simulink model "main_RI_LIEKF"  (R2023a)
settings: Solver=FixedStepAuto  StartTime=0.0  StopTime=220  FixedStep=0.01  RelTol=1e-3
InitFcn:
  | initNavigation0612_AOA;
values from neighbouring files (symbols this model uses):
  CF_enable = 0    [initNavigation.m]
  dt = 0.01    [initNavigation.m]
  dtDelay = -0.03    [initNavigation.m]
  g0 = 9.795    [initNavigation.m]
  gam0_rad = 0/57.3    (= 0)    [initNavigation.m]
  H_sensor_type = 0    [initNavigation.m]
  KF_enable = 1    [initNavigation.m]
  P0 = diag([1*ones(3,1);0.01*ones(3,1);0.1*ones(3,1);0.001*ones(3,1);0.00001*ones(3,1)])    [initNavigation.m]
  P0_RIEKF = diag([1*ones(3,1);0.01*ones(3,1);0.1*ones(3,1);0.001*ones(3,1);0.00001*ones(3,1);      0.01*ones(3,1);[0;2;2]/57.3;[0.1;0.1;0.1]])^2    [initNavigation.m]
  pd0 = 0    [initNavigation.m]
  pe0 = 0    [initNavigation.m]
  phi0_rad = 0/57.3    (= 0)    [initNavigation.m]
  pn0 = 0    [initNavigation.m]
  psi = -178    [initNavigation.m]
  psi0_rad = 0/57.3    (= 0)    [initNavigation.m]
  state_dim = 24    [initNavigation.m]
  Time = 0:0.01:(size(traindata.AttackAngle,1) - 1)*0.01    [NNLiftCoefficientFit.m]
  vd0 = 0    [initNavigation.m]
  ve0 = 0    [initNavigation.m]
  vn0 = 0    [initNavigation.m]
undefined symbols (not defined in the file or in its folder): DiscIntNeverNeededParam, Discrete, INS_CONST, INS_EXPORT, INS_PARAM, magnitude, p, param, pInitialization, sys
libraries: simulink x69, simulink_extras x64, dspstat3 x56, sharedtransform x49, ctrlSharedLib x36, sharedTrackingLibrary x17, FMT_Model_Lib x13, matrix_library x12, deeplib x4, dspsolvers x4, vrlib x4, aerolibconvert2 x1
(part 8 of 22)

== system main_RI_LIEKF/State estimation/0609bk/INS propogation/Init_PVQ ==
  QGC_sensor_reinit : Inport
  accl_B_m/s2_LPF : Inport  Port=2
  Magn_B_guess_LPF : Inport  Port=3
  pos_NED : Inport  Port=4
  vel_NED : Inport  Port=5
  Constant : Constant  Value=[1 0 0 0]  OutDataTypeStr=single
  Constant1 : Constant  OutDataTypeStr=uint8
  Constant2 : Constant  Value=[0;0;0]  OutDataTypeStr=single
  Constant3 : Constant  Value=[0;0;0]  OutDataTypeStr=single
  Detect Increase : simulink/Logic and Bit Operations/Detect Increase  vinit=0.0  OutDataTypeStr=boolean
  Horizontal_attitude : Subsystem  TreatAsAtomicUnit=on
  Memory : Memory
  Scope : Scope  NumInputPorts=2
  Scope1 : Scope
  Scope2 : Scope
  Subsystem : Subsystem
  Subsystem1 : Subsystem
  Switch{,1..3} (4 alike) : Switch  Criteria=u2 > Threshold  SaturateOnIntegerOverflow=off  InputSameDT=off
  quat_0 : Outport
  v0 : Outport  Port=2
  p0 : Outport  Port=3
  wires:
  vel_NED/1 -> Switch2/1
  pos_NED/1 -> Switch3/1
  Switch3/1 -> p0/1
  Switch2/1 -> v0/1
  Constant3/1 -> Switch3/3
  Constant2/1 -> Switch2/3
  Detect Increase/1 -> Scope/2, Switch1/2, Horizontal_attitude/Enable
  Magn_B_guess_LPF/1 -> Subsystem1/1(data)
  QGC_sensor_reinit/1 -> Scope/1, Detect Increase/1
  accl_B_m/s2_LPF/1 -> Subsystem/1(data)
  Switch1/1 -> Scope1/1, Switch/2, Switch3/2, Switch2/2, Memory/1
  Constant1/1 -> Switch1/1
  Constant/1 -> Switch/3
  Horizontal_attitude/1(quat_0) -> Switch/1
  Switch/1 -> Scope2/1, quat_0/1
  Memory/1 -> Switch1/3
  Subsystem/1(mean_data) -> Horizontal_attitude/1(accl_mean_B_m/s_LPF)
  Subsystem1/1(mean_data) -> Horizontal_attitude/2(Magn_mean_B_guess_LPF)

== system main_RI_LIEKF/State estimation/0609bk/INS propogation/att_update ==
  Rbn : Inport
  gyro : Inport  Port=2
  quat_0 : Inport  Port=3  PortDimensions=4
  init_flag : Inport  Port=4
  Bus Creator1 : BusCreator  Inputs=1
  Constant : Constant  Value=dt
  Data Type Conversion : DataTypeConversion  OutDataTypeStr=single  SaturateOnIntegerOverflow=off  RndMeth=Floor
  Delay1 : Delay  DelayLength=1  InitialConditionSource=Input port  InitialCondition=0  ExternalReset=Level hold
      settings: InputPortMap=u0,r5,p4
  Detect Increase : simulink/Logic and Bit Operations/Detect Increase  vinit=0.0  OutDataTypeStr=boolean
  MATLAB Function : MATLAB Function  TreatAsAtomicUnit=on
  Quaternions to Direction Cosine Matrix : sharedtransform/Quaternions to  Direction Cosine Matrix  aMode=aMode
      settings: LibrarySourceBlock=|
      | aerolibtransform2/Quaternions to
      | Direction Cosine Matrix
  Transpose : Math  Operator=transpose
  att_update1 : Outport
  wires:
  init_flag/1 -> Detect Increase/1
  quat_0/1 -> Quaternions to Direction Cosine Matrix/1
  gyro/1 -> MATLAB Function/2(w)  "w"
  Constant/1 -> MATLAB Function/3(dt)
  Quaternions to Direction Cosine Matrix/1 -> Transpose/1
  Transpose/1 -> Delay1/3
  Delay1/1 -> MATLAB Function/1(Rbn_k_1)
  Detect Increase/1 -> Delay1/2
  Bus Creator1/1 -> att_update1/1
  MATLAB Function/1(Rbn) -> Data Type Conversion/1  "DCM_b_n"
  Rbn/1 -> Delay1/1
  Data Type Conversion/1 -> Bus Creator1/1  "DCM_b_n"

== system main_RI_LIEKF/State estimation/0609bk/INS propogation/vel_pos_update ==
  <DCM_b_n> : Inport
  Ab : Inport  Port=2
  v0 : Inport  Port=3
  p0 : Inport  Port=4
  QGC_init : Inport  Port=5
  pn : Inport  Port=6
  vn : Inport  Port=7
  Kinematic Equation : Subsystem
  QGC_init1 : InportShadow  Port=5
  pos update : Subsystem
  vel update : Subsystem
  p_k : Outport
  V : Outport  Port=2
  wires:
  QGC_init1/1 -> pos update/3(QGC_init)
  pos update/1(p_k) -> p_k/1
  p0/1 -> pos update/4(p0)
  pn/1 -> pos update/2(pn)
  v0/1 -> vel update/4(v0)
  vn/1 -> vel update/3(vn)
  Kinematic Equation/1(An) -> vel update/2(An)
  QGC_init/1 -> vel update/1(QGC_init)
  Ab/1 -> Kinematic Equation/2(Ab)
  <DCM_b_n>/1 -> Kinematic Equation/1(Cbn)
  vel update/1(vel_k) -> V/1, pos update/1(vel_k)

== system main_RI_LIEKF/State estimation/15dim KF1/Error State Kalman Filter/Cal Phi ==
  <DCM_b_n> : Inport
  wxyz : Inport  Port=2
  axyz : Inport  Port=3
  Constant : Constant  Value=dt
  MATLAB Function1 : MATLAB Function  TreatAsAtomicUnit=on
  Transpose : Math  Operator=transpose
  Phi : Outport
  wires:
  Transpose/1 -> MATLAB Function1/2(Cnb)
  Constant/1 -> MATLAB Function1/4(dt)
  axyz/1 -> MATLAB Function1/1(axyz)
  wxyz/1 -> MATLAB Function1/3(wxyz)
  MATLAB Function1/1(Phi) -> Phi/1
  <DCM_b_n>/1 -> Transpose/1

== system main_RI_LIEKF/State estimation/15dim KF1/Error State Kalman Filter/Cal Q ==
  <DCM_b_n> : Inport
  wxyz : Inport  Port=2
  Constant : Constant  Value=dt
  MATLAB Function1 : MATLAB Function  TreatAsAtomicUnit=on
  Transpose : Math  Operator=transpose
  Qd : Outport
  wires:
  Transpose/1 -> MATLAB Function1/1(Cnb)
  Constant/1 -> MATLAB Function1/3(dt)
  <DCM_b_n>/1 -> Transpose/1
  MATLAB Function1/1(Qd) -> Qd/1
  wxyz/1 -> MATLAB Function1/2(wxyz)

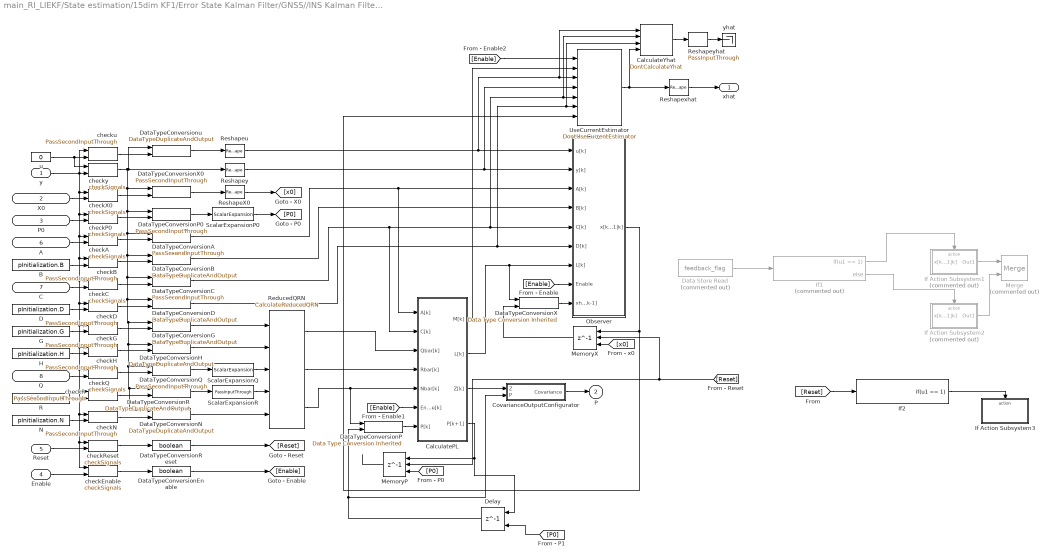
== system main_RI_LIEKF/State estimation/15dim KF1/Error State Kalman Filter/GNSS//INS Kalman Filter1 ==
  y : Inport
  X0 : Inport  Port=2
  P0 : Inport  Port=3
  Enable : Inport  Port=4
  Reset : Inport  Port=5
  A : Inport  Port=6
  C : Inport  Port=7
  Q : Inport  Port=8
  B : Constant  Value=pInitialization.B  VectorParams1D=off  OutDataTypeStr=Inherit: Inherit via back propagation
  CalculatePL : Subsystem  AncestorBlock=ctrlSharedLib/KalmanFilterUtilities/DTCalculatePL  TreatAsAtomicUnit=on  SystemSampleTime=pInitialization.Ts  mask(ctrlKalmanFilterDTCalculatePL){}
      settings: LibrarySourceBlock=ctrlSharedLib/KalmanFilterUtilities/DTCalculatePL
  CalculateYhat : ctrlSharedLib/KalmanFilterUtilities/DontCalculateYhat  SystemSampleTime=-1  VariantActivationTime=update diagram  Latency=0  AutoFrameSizeCalculation=off
  CovarianceOutputConfigurator : Subsystem
  D : Constant  Value=pInitialization.D  VectorParams1D=off  OutDataTypeStr=Inherit: Inherit via back propagation
  Data Store Read : DataStoreRead  Commented=on  DataStoreName=feedback_flag  IndexOptions=Index vector (dialog)  Indices=1  OutputSizes=1
  DataTypeConversionA : ctrlSharedLib/KalmanFilterUtilities/PassSecondInputThrough  SystemSampleTime=-1  VariantActivationTime=update diagram  Latency=0  AutoFrameSizeCalculation=off
  DataTypeConversionB : ctrlSharedLib/Utilities/DataTypeDuplicateAndOutput  SystemSampleTime=-1  VariantActivationTime=update diagram  Latency=0  AutoFrameSizeCalculation=off
  DataTypeConversionC : ctrlSharedLib/KalmanFilterUtilities/PassSecondInputThrough  SystemSampleTime=-1  VariantActivationTime=update diagram  Latency=0  AutoFrameSizeCalculation=off
  DataTypeConversionD : ctrlSharedLib/Utilities/DataTypeDuplicateAndOutput  SystemSampleTime=-1  VariantActivationTime=update diagram  Latency=0  AutoFrameSizeCalculation=off
  DataTypeConversionEnable : DataTypeConversion  OutDataTypeStr=boolean  SaturateOnIntegerOverflow=off  RndMeth=Floor
  DataTypeConversionG : ctrlSharedLib/Utilities/DataTypeDuplicateAndOutput  SystemSampleTime=-1  VariantActivationTime=update diagram  Latency=0  AutoFrameSizeCalculation=off
  DataTypeConversionH : ctrlSharedLib/Utilities/DataTypeDuplicateAndOutput  SystemSampleTime=-1  VariantActivationTime=update diagram  Latency=0  AutoFrameSizeCalculation=off
  DataTypeConversionN : ctrlSharedLib/Utilities/DataTypeDuplicateAndOutput  SystemSampleTime=-1  VariantActivationTime=update diagram  Latency=0  AutoFrameSizeCalculation=off
  DataTypeConversionP : simulink/Signal Attributes/Data Type Conversion Inherited  ConvertRealWorld=Real World Value  DoSatur=off
  DataTypeConversionP0 : ctrlSharedLib/KalmanFilterUtilities/PassSecondInputThrough  SystemSampleTime=-1  VariantActivationTime=update diagram  Latency=0  AutoFrameSizeCalculation=off
  DataTypeConversionQ : ctrlSharedLib/KalmanFilterUtilities/PassSecondInputThrough  SystemSampleTime=-1  VariantActivationTime=update diagram  Latency=0  AutoFrameSizeCalculation=off
  DataTypeConversionR : ctrlSharedLib/Utilities/DataTypeDuplicateAndOutput  SystemSampleTime=-1  VariantActivationTime=update diagram  Latency=0  AutoFrameSizeCalculation=off
  DataTypeConversionReset : DataTypeConversion  OutDataTypeStr=boolean  SaturateOnIntegerOverflow=off  RndMeth=Floor
  DataTypeConversionX : simulink/Signal Attributes/Data Type Conversion Inherited  ConvertRealWorld=Real World Value  DoSatur=off
  DataTypeConversionX0 : ctrlSharedLib/KalmanFilterUtilities/PassSecondInputThrough  SystemSampleTime=-1  VariantActivationTime=update diagram  Latency=0  AutoFrameSizeCalculation=off
  DataTypeConversionu : ctrlSharedLib/Utilities/DataTypeDuplicateAndOutput  SystemSampleTime=-1  VariantActivationTime=update diagram  Latency=0  AutoFrameSizeCalculation=off
  Delay : Delay  DelayLength=1  InitialConditionSource=Input port  ExternalReset=Rising
      settings: InputPortMap=u0,r5,p4
  G : Constant  Value=pInitialization.G  VectorParams1D=off  OutDataTypeStr=Inherit: Inherit via back propagation
  H : Constant  Value=pInitialization.H  VectorParams1D=off  OutDataTypeStr=Inherit: Inherit via back propagation
  If Action Subsystem1 : Subsystem  Commented=on  TreatAsAtomicUnit=on
  If Action Subsystem2 : Subsystem  Commented=on  TreatAsAtomicUnit=on
  If Action Subsystem3 : Subsystem  TreatAsAtomicUnit=on
  If1 : If  Commented=on  IfExpression=u1 == 1
  If2 : If  IfExpression=u1 == 1  ShowElse=off
  MemoryP : Delay  DelayLength=1  InitialConditionSource=Input port  ExternalReset=Rising  SampleTime=pInitialization.Ts
      settings: InputPortMap=u0,r5,p4
  MemoryX : Delay  DelayLength=1  InitialConditionSource=Input port  ExternalReset=Rising  SampleTime=pInitialization.Ts
      settings: InputPortMap=u0,r5,p4
  Merge : Merge  Commented=on
  N : Constant  Value=pInitialization.N  VectorParams1D=off  OutDataTypeStr=Inherit: Inherit via back propagation
  Observer : Subsystem
  R : Constant  Value=pInitialization.R  VectorParams1D=off  OutDataTypeStr=Inherit: Inherit via back propagation
  ReducedQRN : ctrlSharedLib/KalmanFilterUtilities/CalculateReducedQRN  SystemSampleTime=-1  VariantActivationTime=update diagram  Latency=0  AutoFrameSizeCalculation=off
  ReshapeX0 : Reshape
  Reshapeu : Reshape
  Reshapexhat : Reshape
  Reshapey : Reshape
  Reshapeyhat : ctrlSharedLib/Utilities/PassInputThrough  SystemSampleTime=-1  VariantActivationTime=update diagram  Latency=0  AutoFrameSizeCalculation=off
  ScalarExpansionP0 : ctrlSharedLib/Utilities/ScalarExpansion  n=pInitialization.Ns  IsStrictPositiveDefinite=on  OutputSquareRootY=off
  ScalarExpansionQ : ctrlSharedLib/Utilities/ScalarExpansion  n=pInitialization.Nw  IsStrictPositiveDefinite=off  OutputSquareRootY=off
  ScalarExpansionR : ctrlSharedLib/Utilities/PassInputThrough  SystemSampleTime=-1  VariantActivationTime=update diagram  Latency=0  AutoFrameSizeCalculation=off
  UseCurrentEstimator : ctrlSharedLib/KalmanFilterUtilities/DontUseCurrentEstimator  SystemSampleTime=-1  VariantActivationTime=update diagram  Latency=0  AutoFrameSizeCalculation=off
  checkA : ctrlSharedLib/KalmanFilterUtilities/checkSignals  Ts=pInitialization.Ts  Ns=pInitialization.Ns  Nu=pInitialization.Nu  Nw=pInitialization.Nw  Ny=pInitialization.Ny
  checkB : ctrlSharedLib/KalmanFilterUtilities/PassSecondInputThrough  SystemSampleTime=-1  VariantActivationTime=update diagram  Latency=0  AutoFrameSizeCalculation=off
  checkC : ctrlSharedLib/KalmanFilterUtilities/checkSignals  Ts=pInitialization.Ts  Ns=pInitialization.Ns  Nu=pInitialization.Nu  Nw=pInitialization.Nw  Ny=pInitialization.Ny
  checkD : ctrlSharedLib/KalmanFilterUtilities/PassSecondInputThrough  SystemSampleTime=-1  VariantActivationTime=update diagram  Latency=0  AutoFrameSizeCalculation=off
  checkEnable : ctrlSharedLib/KalmanFilterUtilities/checkSignals  Ts=pInitialization.Ts  Ns=pInitialization.Ns  Nu=pInitialization.Nu  Nw=pInitialization.Nw  Ny=pInitialization.Ny
  checkG : ctrlSharedLib/KalmanFilterUtilities/PassSecondInputThrough  SystemSampleTime=-1  VariantActivationTime=update diagram  Latency=0  AutoFrameSizeCalculation=off
  checkH : ctrlSharedLib/KalmanFilterUtilities/PassSecondInputThrough  SystemSampleTime=-1  VariantActivationTime=update diagram  Latency=0  AutoFrameSizeCalculation=off
  checkN : ctrlSharedLib/KalmanFilterUtilities/PassSecondInputThrough  SystemSampleTime=-1  VariantActivationTime=update diagram  Latency=0  AutoFrameSizeCalculation=off
  checkP0 : ctrlSharedLib/KalmanFilterUtilities/checkSignals  Ts=pInitialization.Ts  Ns=pInitialization.Ns  Nu=pInitialization.Nu  Nw=pInitialization.Nw  Ny=pInitialization.Ny
  checkQ : ctrlSharedLib/KalmanFilterUtilities/checkSignals  Ts=pInitialization.Ts  Ns=pInitialization.Ns  Nu=pInitialization.Nu  Nw=pInitialization.Nw  Ny=pInitialization.Ny
  checkR : ctrlSharedLib/KalmanFilterUtilities/PassSecondInputThrough  SystemSampleTime=-1  VariantActivationTime=update diagram  Latency=0  AutoFrameSizeCalculation=off
  checkReset : ctrlSharedLib/KalmanFilterUtilities/checkSignals  Ts=pInitialization.Ts  Ns=pInitialization.Ns  Nu=pInitialization.Nu  Nw=pInitialization.Nw  Ny=pInitialization.Ny
  checkX0 : ctrlSharedLib/KalmanFilterUtilities/checkSignals  Ts=pInitialization.Ts  Ns=pInitialization.Ns  Nu=pInitialization.Nu  Nw=pInitialization.Nw  Ny=pInitialization.Ny
  checku : ctrlSharedLib/KalmanFilterUtilities/PassSecondInputThrough  SystemSampleTime=-1  VariantActivationTime=update diagram  Latency=0  AutoFrameSizeCalculation=off
  checky : ctrlSharedLib/KalmanFilterUtilities/checkSignals  Ts=pInitialization.Ts  Ns=pInitialization.Ns  Nu=pInitialization.Nu  Nw=pInitialization.Nw  Ny=pInitialization.Ny
  u : Constant  Value=0  OutDataTypeStr=Inherit: Inherit via back propagation
  yhat : Terminator
  xhat : Outport  VectorParamsAs1DForOutWhenUnconnected=off
  P : Outport  Port=2
  wires:
  If2/1 -> If Action Subsystem3/Action
  [Reset] -> If2/1
  MemoryP/1 -> ?
  Observer/1(x[k+1|k]) -> MemoryX/1, UseCurrentEstimator/7
  [Reset] -> MemoryP/2, MemoryX/2
  If Action Subsystem2/1(Out1) -> Merge/2
  If Action Subsystem1/1(Out1) -> Merge/1
  If1/2 -> If Action Subsystem2/Action
  If1/1 -> If Action Subsystem1/Action
  Data Store Read/1 -> If1/1
  [P0] -> Delay/3
  CalculatePL/3(Z[k]) -> CovarianceOutputConfigurator/1(Z)
  Reshapexhat/1 -> xhat/1
  Reshapeyhat/1 -> yhat/1
  UseCurrentEstimator/1 -> Reshapexhat/1, CalculateYhat/4
  checku/1 -> DataTypeConversionu/2
  DataTypeConversionu/1 -> Reshapeu/1
  CovarianceOutputConfigurator/1(Covariance) -> P/1
  DataTypeConversionC/1 -> Observer/5(C[k]), UseCurrentEstimator/5, CalculateYhat/2, CalculatePL/2(C[k])
  ScalarExpansionR/1 -> ReducedQRN/4
  ScalarExpansionQ/1 -> ReducedQRN/3
  ScalarExpansionP0/1 -> [P0]
  CalculatePL/4(P[k+1]) -> MemoryP/1, Delay/1
  DataTypeConversionReset/1 -> [Reset]
  checkReset/1 -> DataTypeConversionReset/1
  checky/1 -> DataTypeConversionX0/1, DataTypeConversionP0/1, DataTypeConversionC/1, DataTypeConversionD/1, DataTypeConversionG/1, DataTypeConversionH/1, DataTypeConversionQ/1, DataTypeConversionR/1, DataTypeConversionN/1, DataTypeConversionB/1, DataTypeConversionA/1, Reshapey/1, DataTypeConversionu/1
  ReshapeX0/1 -> [x0]
  Delay/1 -> CovarianceOutputConfigurator/2(P), DataTypeConversionP/2
  [P0] -> MemoryP/3
  CalculateYhat/1 -> Reshapeyhat/1
  [Enable] -> UseCurrentEstimator/1
  CalculatePL/1(M[k]) -> UseCurrentEstimator/2
  CalculatePL/2(L[k]) -> Observer/7(L[k]), DataTypeConversionX/1
  Reshapey/1 -> Observer/2(y[k]), UseCurrentEstimator/4
  Reshapeu/1 -> Observer/1(u[k]), UseCurrentEstimator/3, CalculateYhat/1
  y/1 -> checky/2, checku/1, checkX0/1, checkP0/1, checkA/1, checkB/1, checkC/1, checkD/1, checkG/1, checkH/1, checkQ/1, checkR/1, checkN/1, checkReset/1, checkEnable/1
  u/1 -> checku/2, checky/1
  DataTypeConversionP/1 -> CalculatePL/7(P[k])
  [Enable] -> Observer/8(Enable)
  DataTypeConversionX/1 -> Observer/9(xhat[k|k-1])
  DataTypeConversionX0/1 -> ReshapeX0/1
  [x0] -> MemoryX/3
  X0/1 -> checkX0/2
  DataTypeConversionD/1 -> Observer/6(D[k]), UseCurrentEstimator/6, CalculateYhat/3
  DataTypeConversionB/1 -> Observer/4(B[k])
  DataTypeConversionA/1 -> Observer/3(A[k]), CalculatePL/1(A[k])
  checkB/1 -> DataTypeConversionB/2
  B/1 -> checkB/2
  ReducedQRN/3 -> CalculatePL/5(Nbar[k]), DataTypeConversionP/1
  ReducedQRN/2 -> CalculatePL/4(Rbar[k])
  ReducedQRN/1 -> CalculatePL/3(Qbar[k])
  checkA/1 -> DataTypeConversionA/2
  A/1 -> checkA/2
  [Enable] -> CalculatePL/6(Enable[k])
  DataTypeConversionEnable/1 -> [Enable]
  checkEnable/1 -> DataTypeConversionEnable/1
  Enable/1 -> checkEnable/2
  DataTypeConversionP0/1 -> ScalarExpansionP0/1
  Reset/1 -> checkReset/2
  DataTypeConversionN/1 -> ReducedQRN/5
  checkN/1 -> DataTypeConversionN/2
  checkR/1 -> DataTypeConversionR/2
  DataTypeConversionR/1 -> ScalarExpansionR/1
  checkQ/1 -> DataTypeConversionQ/2
  DataTypeConversionQ/1 -> ScalarExpansionQ/1
  DataTypeConversionH/1 -> ReducedQRN/2
  checkH/1 -> DataTypeConversionH/2
  DataTypeConversionG/1 -> ReducedQRN/1
  checkG/1 -> DataTypeConversionG/2
  checkD/1 -> DataTypeConversionD/2
  checkC/1 -> DataTypeConversionC/2
  checkP0/1 -> DataTypeConversionP0/2
  checkX0/1 -> DataTypeConversionX0/2
  MemoryX/1 -> DataTypeConversionX/2
  N/1 -> checkN/2
  R/1 -> checkR/2
  Q/1 -> checkQ/2
  H/1 -> checkH/2
  G/1 -> checkG/2
  D/1 -> checkD/2
  P0/1 -> checkP0/2
  C/1 -> checkC/2

== system main_RI_LIEKF/State estimation/15dim KF1/Error State Kalman Filter/Subsystem ==
  data : Inport
  Detect Change : simulink/Logic and Bit Operations/Detect Change  vinit=0  InputProcessing=Columns as channels (frame based)  OutDataTypeStr=boolean
  Selector : Selector  InputPortWidth=3  IndexOptions=Index vector (dialog)  Indices=[3]  OutputSizes=1
  Zero-Order Hold : ZeroOrderHold  SampleTime=0.1
  Zero-Order Hold1 : ZeroOrderHold  SampleTime=0.01
  flag : Outport
  wires:
  Zero-Order Hold1/1 -> Detect Change/1
  Detect Change/1 -> flag/1
  Selector/1 -> Zero-Order Hold1/1
  data/1 -> Zero-Order Hold/1
  Zero-Order Hold/1 -> Selector/1

== system main_RI_LIEKF/State estimation/15dim KF1/INS propogation/Init_PVQ2 ==
  QGC_sensor_reinit : Inport
  accl_B_m/s2_LPF : Inport  Port=2
  Magn_B_guess_LPF : Inport  Port=3
  pos_NED : Inport  Port=4
  vel_NED : Inport  Port=5
  Constant : Constant  Value=[0 0 0 1]  OutDataTypeStr=single
  Constant1 : Constant  OutDataTypeStr=uint8
  Constant2 : Constant  Value=[0;0;0]  OutDataTypeStr=single
  Constant3 : Constant  Value=[0;0;0]  OutDataTypeStr=single
  Detect Increase : simulink/Logic and Bit Operations/Detect Increase  vinit=0.0  OutDataTypeStr=boolean
  Horizontal_attitude : Subsystem  TreatAsAtomicUnit=on
  Memory : Memory
  Scope : Scope  NumInputPorts=2
  Scope1 : Scope
  Scope2 : Scope
  Subsystem : Subsystem
  Subsystem1 : Subsystem
  Switch{,1..3} (4 alike) : Switch  Criteria=u2 > Threshold  SaturateOnIntegerOverflow=off  InputSameDT=off
  quat_0 : Outport
  v0 : Outport  Port=2
  p0 : Outport  Port=3
  wires:
  Subsystem1/1(mean_data) -> Horizontal_attitude/2(Magn_mean_B_guess_LPF)
  Subsystem/1(mean_data) -> Horizontal_attitude/1(accl_mean_B_m/s_LPF)
  Memory/1 -> Switch1/3
  Horizontal_attitude/1(quat_0) -> Switch/1
  Constant/1 -> Switch/3
  Constant1/1 -> Switch1/1
  Switch1/1 -> Memory/1, Switch2/2, Switch3/2, Switch/2, Scope1/1
  accl_B_m/s2_LPF/1 -> Subsystem/1(data)
  QGC_sensor_reinit/1 -> Detect Increase/1, Scope/1
  Magn_B_guess_LPF/1 -> Subsystem1/1(data)
  Detect Increase/1 -> Horizontal_attitude/Enable, Switch1/2, Scope/2
  Constant2/1 -> Switch2/3
  Constant3/1 -> Switch3/3
  Switch2/1 -> v0/1
  Switch3/1 -> p0/1
  pos_NED/1 -> Switch3/1
  vel_NED/1 -> Switch2/1
  Switch/1 -> Scope2/1, quat_0/1

== system main_RI_LIEKF/State estimation/15dim KF1/INS propogation/accl bias compensation ==
  raw <accl_B_m/s2_LPF> : Inport
  dda : Inport  Port=2
  Add2 : Sum
  Data Type Conversion6 : DataTypeConversion  OutDataTypeStr=single  SaturateOnIntegerOverflow=off  RndMeth=Floor
  error compensation1 : Subsystem
  fb : Outport
  da : Outport  Port=2
  wires:
  dda/1 -> error compensation1/1(dda)
  raw <accl_B_m/s2_LPF>/1 -> Add2/1
  Data Type Conversion6/1 -> fb/1
  Add2/1 -> Data Type Conversion6/1
  error compensation1/1(da) -> Add2/2, da/1

== system main_RI_LIEKF/State estimation/15dim KF1/INS propogation/att_update ==
  dtheta : Inport
  gyro : Inport  Port=2
  quat_0 : Inport  Port=3  PortDimensions=4
  init_flag : Inport  Port=4
  Bus Creator : BusCreator  Inputs=2
  Data Type Conversion1 : DataTypeConversion  OutDataTypeStr=single  SaturateOnIntegerOverflow=off  RndMeth=Floor
  Data Type Conversion2 : DataTypeConversion  OutDataTypeStr=single  SaturateOnIntegerOverflow=off  RndMeth=Floor
  Data Type Conversion3 : DataTypeConversion  OutDataTypeStr=double  SaturateOnIntegerOverflow=off  RndMeth=Floor
  Data Type Conversion4 : DataTypeConversion  OutDataTypeStr=double  SaturateOnIntegerOverflow=off  RndMeth=Floor
  Delay : Delay  DelayLength=1  InitialConditionSource=Input port  ExternalReset=Level hold
      settings: InputPortMap=u0,r5,p4
  Detect Increase : simulink/Logic and Bit Operations/Detect Increase  vinit=0.0  OutDataTypeStr=boolean
  Gain : Gain  Gain=dt  OutDataTypeStr=double
  Gain1 : Gain  Gain=-1
  JPLQuatMult : MATLAB Function  TreatAsAtomicUnit=on
  JPLQuatMult1 : MATLAB Function  TreatAsAtomicUnit=on
  JPLrv2q : MATLAB Function  TreatAsAtomicUnit=on
  JPLrv2q1 : MATLAB Function  TreatAsAtomicUnit=on
  MATLAB Function1 : MATLAB Function  TreatAsAtomicUnit=on
  Scope : Scope
  Transpose1 : Math  Operator=transpose  SignedPower=on
  att_update : Outport
  wires:
  Gain1/1 -> Data Type Conversion4/1, Scope/1
  JPLQuatMult1/1(q_t) -> Data Type Conversion3/1  "q_update"
  JPLQuatMult/1(q_t) -> JPLQuatMult1/2(quatB)  "q_update"
  dtheta/1 -> Gain1/1
  JPLrv2q1/1(updateQuat) -> JPLQuatMult1/1(quatA)
  Data Type Conversion4/1 -> JPLrv2q1/1(deltaTheta)  "q_update"
  Transpose1/1 -> Bus Creator/2  "DCM_b_n"
  gyro/1 -> Gain/1
  Data Type Conversion3/1 -> Data Type Conversion1/1, Delay/1, MATLAB Function1/1(q)  "q_update"
  Data Type Conversion1/1 -> Bus Creator/1  "q_update"
  JPLrv2q/1(quaternion) -> JPLQuatMult/1(quatA)
  Gain/1 -> JPLrv2q/1(rotVec)  "correctedDelAng"
  Delay/1 -> JPLQuatMult/2(quatB)
  quat_0/1 -> Delay/3
  MATLAB Function1/1(Rot) -> Data Type Conversion2/1
  Data Type Conversion2/1 -> Transpose1/1  "DCM_n_b"
  Bus Creator/1 -> att_update/1
  init_flag/1 -> Detect Increase/1
  Detect Increase/1 -> Delay/2

== system main_RI_LIEKF/State estimation/15dim KF1/INS propogation/gyro bias compensation ==
  raw <gyro_B_rad/s_LPF> : Inport
  ddg : Inport  Port=2
  Measuemrnt Enable Flag : Inport  Port=3
  Add1 : Sum
  Data Type Conversion4 : DataTypeConversion  OutDataTypeStr=single  SaturateOnIntegerOverflow=off  RndMeth=Floor
  Scope1 : Scope
  error compensation : Subsystem
  wb : Outport
  dg : Outport  Port=2
  wires:
  Data Type Conversion4/1 -> wb/1
  raw <gyro_B_rad/s_LPF>/1 -> Add1/1
  error compensation/1(dg) -> Scope1/1, dg/1, Add1/2
  Measuemrnt Enable Flag/1 -> error compensation/2(Enable)
  Add1/1 -> Data Type Conversion4/1
  ddg/1 -> error compensation/1(ddg)

== system main_RI_LIEKF/State estimation/15dim KF1/INS propogation/vel_pos_update ==
  <DCM_b_n> : Inport
  Ab : Inport  Port=2
  v0 : Inport  Port=3
  p0 : Inport  Port=4
  QGC_init : Inport  Port=5
  dp : Inport  Port=6
  dv : Inport  Port=7
  Kinematic Equation : Subsystem
  QGC_init1 : InportShadow  Port=5
  pos update : Subsystem
  vel update : Subsystem
  p_k : Outport
  V : Outport  Port=2
  wires:
  QGC_init1/1 -> pos update/3(QGC_init)
  pos update/1(p_k) -> p_k/1
  p0/1 -> pos update/4(p0)
  dp/1 -> pos update/2(dp)
  v0/1 -> vel update/4(v0)
  dv/1 -> vel update/3(KFState_dv)
  Kinematic Equation/1(An) -> vel update/2(An)
  QGC_init/1 -> vel update/1(QGC_init)
  vel update/1(vel_k) -> pos update/1(vel_k), V/1
  Ab/1 -> Kinematic Equation/2(Ab)
  <DCM_b_n>/1 -> Kinematic Equation/1(Cbn)

== system main_RI_LIEKF/State estimation/15dim KF1/Subsystem2/Measurement Update ==
  note: Xk/k-1=FXk-1
      | Xk=Xk/k-1+K(Z-HXk/k-1)
      | K=Pk/k-1H(HPk/k-1H+Rk)-1
      | Pk/k-1=FPk-1F+GQG
      | Pk=(I-KH)Pk/k-1
  note: 计算卡尔曼增益Kk
  Z : Inport
  H : Inport  Port=2
  R : Inport  Port=3
  Xk_k_1 : Inport  Port=4
  Pk_k_1 : Inport  Port=5
  Enable : EnablePort
  Add1 : Sum
  Add2 : Sum
  Add3 : Sum  Inputs=+-
  Add4 : Sum  Inputs=+-
  Constant : Constant  Value=eye(15)  OutDataTypeStr=single
  Math Function1 : Math  Operator=transpose  SignedPower=on
  Math Function2 : Math  Operator=transpose  SignedPower=on
  MatrixMultiply2 : Product  Inputs=3  Multiplication=Matrix(*)
  MatrixMultiply3 : Product  Inputs=3  Multiplication=Matrix(*)
  MatrixMultiply{4..7} (4 alike) : Product  Multiplication=Matrix(*)
  Product : Product  Inputs=/  Multiplication=Matrix(*)
  Xk : Outport
  Pk : Outport  Port=2
  wires:
  Xk_k_1/1 -> [Xk_k_1]
  Add2/1 -> Xk/1
  Pk_k_1/1 -> [Pk_k_1]
  R/1 -> [R]
  [H] -> MatrixMultiply6/2
  Add3/1 -> MatrixMultiply4/2
  [Pk_k_1] -> MatrixMultiply3/2
  Constant/1 -> Add4/1
  MatrixMultiply6/1 -> Add4/2
  [Kk] -> MatrixMultiply6/1
  [H] -> Math Function2/1
  Math Function2/1 -> MatrixMultiply3/3
  [H] -> Math Function1/1
  [R] -> Add1/2
  MatrixMultiply2/1 -> [Kk]
  [Xk_k_1] -> MatrixMultiply5/2
  Add4/1 -> MatrixMultiply7/1
  [Xk_k_1] -> Add2/1
  Add1/1 -> Product/1
  MatrixMultiply7/1 -> Pk/1
  Z/1 -> [Z]
  Product/1 -> MatrixMultiply2/3
  MatrixMultiply4/1 -> Add2/2
  [Z] -> Add3/1
  [Pk_k_1] -> MatrixMultiply7/2
  Math Function1/1 -> MatrixMultiply2/2
  MatrixMultiply5/1 -> Add3/2
  MatrixMultiply3/1 -> Add1/1
  [Pk_k_1] -> MatrixMultiply2/1
  [H] -> MatrixMultiply5/1
  [Kk] -> MatrixMultiply4/1
  H/1 -> [H]
  [H] -> MatrixMultiply3/1

== system main_RI_LIEKF/State estimation/15dim KF1/Subsystem2/Time Update ==
  F : Inport
  Q : Inport  Port=2
  P : Inport  Port=3
  X : Inport  Port=4
  Add : Sum
  Math Function3 : Math  Operator=transpose  SignedPower=on
  MatrixMultiply : Product  Multiplication=Matrix(*)
  MatrixMultiply1 : Product  Inputs=3  Multiplication=Matrix(*)
  Xk/k_1 : Outport
  Pk/k_1 : Outport  Port=2
  wires:
  P/1 -> [P]
  MatrixMultiply/1 -> Xk/k_1/1
  F/1 -> [F]
  Q/1 -> [Q]
  Math Function3/1 -> MatrixMultiply1/3
  [P] -> MatrixMultiply1/2
  Add/1 -> Pk/k_1/1
  [X] -> MatrixMultiply/2
  MatrixMultiply1/1 -> Add/1
  [F] -> MatrixMultiply/1
  X/1 -> [X]
  [F] -> MatrixMultiply1/1
  [F] -> Math Function3/1
  [Q] -> Add/2

== system main_RI_LIEKF/State estimation/ER EKF/Error State Kalman Filter/Cal Q1 ==
  Constant : Constant  Value=dt  OutDataTypeStr=double
  MATLAB Function1 : MATLAB Function  TreatAsAtomicUnit=on
  Qd : Outport
  wires:
  MATLAB Function1/1(Q) -> Qd/1
  Constant/1 -> MATLAB Function1/1(dt)

== system main_RI_LIEKF/State estimation/ER EKF/Error State Kalman Filter/Extended Kalman Filter1 ==
  Q : Inport
  Enable1 : Inport  Port=2
  y1 : Inport  Port=3
  R1 : Inport  Port=4
  BlockOrdering : Constant  Value=true()  OutDataTypeStr=boolean
  Correct1 : Subsystem  AncestorBlock=sharedTrackingLibrary/Extras/EKFCorrect  TreatAsAtomicUnit=on  SystemSampleTime=p.SampleTimes.MeasurementFcn(1)  mask(EKFCorrect){ProcessedMaskData=p}
      mask init: same as main_RI_LIEKF/State estimation/0609bk/Error State Kalman Filter/Extended Kalman Filter1/Correct1
      settings: LibrarySourceBlock=sharedTrackingLibrary/Extras/EKFCorrect
  DataStoreMemory - P : DataStoreMemory  DataStoreName=P  InitialValue=p.InitialCovariance  ShowAdditionalParam=off  OutDataTypeStr=p.DataType
  DataStoreMemory - x : DataStoreMemory  DataStoreName=x  InitialValue=p.InitialState  ShowAdditionalParam=off  OutDataTypeStr=p.DataType
  DataTypeConversion_Enable1 : DataTypeConversion  OutDataTypeStr=boolean  SaturateOnIntegerOverflow=off  RndMeth=Floor
  DataTypeConversion_Q : DataTypeConversion  OutDataTypeStr=p.DataType  SaturateOnIntegerOverflow=off  RndMeth=Floor
  DataTypeConversion_R1 : DataTypeConversion  OutDataTypeStr=p.DataType  SaturateOnIntegerOverflow=off  RndMeth=Floor
  DataTypeConversion_uMeas1 : DataTypeConversion  OutDataTypeStr=p.DataType  SaturateOnIntegerOverflow=off  RndMeth=Floor
  DataTypeConversion_uState : DataTypeConversion  OutDataTypeStr=p.DataType  SaturateOnIntegerOverflow=off  RndMeth=Floor
  DataTypeConversion_y1 : DataTypeConversion  OutDataTypeStr=p.DataType  SaturateOnIntegerOverflow=off  RndMeth=Floor
  MeasurementFcn1Inputs : Constant  Value=0  OutDataTypeStr=p.DataType  SampleTime=p.SampleTimes.MeasurementFcn(1)
  Output : Subsystem  TreatAsAtomicUnit=on  SystemSampleTime=p.SampleTimes.Output
  Predict : Subsystem  TreatAsAtomicUnit=on  SystemSampleTime=p.SampleTimes.StateTransitionFcn  mask(EKFPredict){ProcessedMaskData=p}
      mask init: same as main_RI_LIEKF/State estimation/0609bk/Error State Kalman Filter/Extended Kalman Filter1/Predict
  StateTransitionFcnInputs : Constant  Value=0  OutDataTypeStr=p.DataType  SampleTime=p.SampleTimes.StateTransitionFcn
  checkMeasurementFcn1Signals : S-Function  FunctionName=ekfukfCheckSignals  Parameters=signalCheck.BlockPath, signalCheck.MeasurementFcn{1}.PortNames, signalCheck.MeasurementFcn{1}.SampleTime, signalCheck.DataType, signalCheck.MeasurementFcn{1}.PortDimensions, 1, signalCheck.MeasurementFcn{1}.HasAdditiveNoise  SFunctionDeploymentMode=off  EnableBusSupport=off
  checkStateTransitionFcnSignals : S-Function  FunctionName=ekfukfCheckSignals  Parameters=signalCheck.BlockPath, signalCheck.StateTransitionFcn.PortNames, signalCheck.StateTransitionFcn.SampleTime, signalCheck.DataType, signalCheck.StateTransitionFcn.PortDimensions, 0, signalCheck.StateTransitionFcn.HasAdditiveNoise  SFunctionDeploymentMode=off  EnableBusSupport=off
  xhat : Outport  VectorParamsAs1DForOutWhenUnconnected=off
  P : Outport  Port=2
  wires:
  y1/1 -> checkMeasurementFcn1Signals/2, DataTypeConversion_y1/1
  R1/1 -> checkMeasurementFcn1Signals/3, DataTypeConversion_R1/1
  Q/1 -> checkStateTransitionFcnSignals/1, DataTypeConversion_Q/1
  DataTypeConversion_Q/1 -> Predict/1(Q)
  Enable1/1 -> checkMeasurementFcn1Signals/1, DataTypeConversion_Enable1/1
  DataTypeConversion_Enable1/1 -> Correct1/Enable
  Output/2(P) -> P/1
  Output/1(x) -> xhat/1
  StateTransitionFcnInputs/1 -> checkStateTransitionFcnSignals/2, DataTypeConversion_uState/1
  DataTypeConversion_uState/1 -> Predict/2(uState)
  DataTypeConversion_y1/1 -> Correct1/1(yMeas)
  MeasurementFcn1Inputs/1 -> checkMeasurementFcn1Signals/4, DataTypeConversion_uMeas1/1
  DataTypeConversion_R1/1 -> Correct1/2(R)
  DataTypeConversion_uMeas1/1 -> Correct1/3(uMeas)
  BlockOrdering/1 -> [FirstOperation]
  [FirstOperation] -> Correct1/4(uBlockOrdering)
  [AfterCorrect] -> Output/1(uBlockOrdering)
  Output/3(yBlockOrdering) -> [AfterOutput]
  [AfterOutput] -> Predict/3(uBlockOrdering)
  Correct1/1(yBlockOrdering) -> [AfterCorrect]

== system main_RI_LIEKF/State estimation/ER EKF/Error State Kalman Filter/Simulink Function - GPS Measurements ==
  GPSMeasurementFcn : TriggerPort  TriggerType=function-call  IsSimulinkFunction=on  FunctionName=GPSMeasurementFcn  VariantControl=Variant
  Add : Sum
  Constant6 : Constant  Value=[eye(6),zeros(6,9)]  OutDataTypeStr=single
  Product : Product  Multiplication=Matrix(*)
  x : ArgIn  DisableCoverage=on  OutDataTypeStr=single  PortDimensions=15  ArgumentName=x
  v : ArgIn  DisableCoverage=on  Port=2  OutDataTypeStr=single  PortDimensions=6  ArgumentName=v
  y : ArgOut  DisableCoverage=on  OutDataTypeStr=single  PortDimensions=6  ArgumentName=y
  wires:
  Add/1 -> y/1
  Product/1 -> Add/1
  x/1 -> Product/2
  Constant6/1 -> Product/1
  v/1 -> Add/2

== system main_RI_LIEKF/State estimation/ER EKF/Error State Kalman Filter/Simulink Function - GPS Measurements1 ==
  DCM_b_n : Inport
  DynamicMeasurementFcn_Dyn : TriggerPort  TriggerType=function-call  IsSimulinkFunction=on  FunctionName=DynamicMeasurementFcn_Dyn  VariantControl=Variant
  Add : Sum  Commented=on
  Add1 : Sum
  Constant : Constant  Commented=on  Value=dt  OutDataTypeStr=single
  Constant6 : Constant  Value=[zeros(3,3),eye(3),zeros(3,12);zeros(3,15),eye(3)]  OutDataTypeStr=single
  Data Type Conversion6 : DataTypeConversion  Commented=on  OutDataTypeStr=single  SaturateOnIntegerOverflow=off  RndMeth=Floor
  From7 : From  Commented=on  GotoTag=DCM_b_n
  Goto : Goto  Commented=on  GotoTag=DCM_b_n
  MATLAB Function1 : MATLAB Function  Commented=on  TreatAsAtomicUnit=on
  Product : Product  Commented=on  Multiplication=Matrix(*)
  Product1 : Product  Multiplication=Matrix(*)
  x : ArgIn  DisableCoverage=on  OutDataTypeStr=single  PortDimensions=18  ArgumentName=x
  v : ArgIn  DisableCoverage=on  Port=2  OutDataTypeStr=single  PortDimensions=6  ArgumentName=v
  y : ArgOut  DisableCoverage=on  OutDataTypeStr=single  PortDimensions=6  ArgumentName=y
  wires:
  x/1 -> Product1/2
  Constant6/1 -> Product1/1
  Product1/1 -> Add1/1
  v/1 -> Add1/2
  Add1/1 -> y/1
  Data Type Conversion6/1 -> Product/1
  DCM_b_n/1 -> Goto/1
  Constant/1 -> MATLAB Function1/2(dt)
  From7/1 -> MATLAB Function1/1(Cbn)
  MATLAB Function1/1(H) -> Data Type Conversion6/1
  Product/1 -> Add/1

== system main_RI_LIEKF/State estimation/ER EKF/Error State Kalman Filter/Simulink Function - GPS Measurements2 ==
  ZUPTMeasurementFcn2 : TriggerPort  TriggerType=function-call  IsSimulinkFunction=on  FunctionName=ZUPTMeasurementFcn2  VariantControl=Variant
  Add : Sum
  Constant6 : Constant  Value=[zeros(3,3),eye(3),zeros(3,12)]  OutDataTypeStr=single
  Product : Product  Multiplication=Matrix(*)
  x : ArgIn  DisableCoverage=on  OutDataTypeStr=single  PortDimensions=18  ArgumentName=x
  v : ArgIn  DisableCoverage=on  Port=2  OutDataTypeStr=single  PortDimensions=3  ArgumentName=v
  y : ArgOut  DisableCoverage=on  OutDataTypeStr=single  PortDimensions=3  ArgumentName=y
  wires:
  v/1 -> Add/2
  Constant6/1 -> Product/1
  x/1 -> Product/2
  Product/1 -> Add/1
  Add/1 -> y/1

== system main_RI_LIEKF/State estimation/ER EKF/Error State Kalman Filter/Simulink Function - State Transition ==
  DCM_b_n : Inport
  wxyz : Inport  Port=2
  fbxyz : Inport  Port=3
  stateTransitionFcn : TriggerPort  TriggerType=function-call  IsSimulinkFunction=on  FunctionName=stateTransitionFcn  VariantControl=Variant
  Add : Sum
  Cal Phi : Subsystem
  Constant : Constant  Value=0.01  OutDataTypeStr=single
  Data Type Conversion1 : DataTypeConversion  OutDataTypeStr=single  SaturateOnIntegerOverflow=off  RndMeth=Floor
  Data Type Conversion6 : DataTypeConversion  OutDataTypeStr=single  SaturateOnIntegerOverflow=off  RndMeth=Floor
  MATLAB Function : MATLAB Function  TreatAsAtomicUnit=on
  Product1 : Product  Multiplication=Matrix(*)
  Product2 : Product  Multiplication=Matrix(*)
  Transpose : Math  Operator=transpose
  x : ArgIn  DisableCoverage=on  OutDataTypeStr=single  PortDimensions=15  ArgumentName=x
  w : ArgIn  Port=2  OutDataTypeStr=single  PortDimensions=12  ArgumentName=w
  xNext : ArgOut  DisableCoverage=on  OutDataTypeStr=single  PortDimensions=15  ArgumentName=xNext
  wires:
  Data Type Conversion6/1 -> Add/2
  Data Type Conversion1/1 -> Add/1
  Cal Phi/1(Phi) -> Product2/1
  fbxyz/1 -> [fbxyz]
  wxyz/1 -> [wxyz]
  DCM_b_n/1 -> [DCM_b_n]
  Constant/1 -> MATLAB Function/3(dt)
  [wxyz] -> MATLAB Function/2(wxyz)
  Transpose/1 -> MATLAB Function/1(Cnb)
  [DCM_b_n] -> Transpose/1
  [DCM_b_n] -> Cal Phi/1(<DCM_b_n>)
  [wxyz] -> Cal Phi/2(wxyz)
  [fbxyz] -> Cal Phi/3(axyz)
  Add/1 -> xNext/1
  Product1/1 -> Data Type Conversion1/1
  w/1 -> Product1/2
  MATLAB Function/1(G) -> Product1/1
  Product2/1 -> Data Type Conversion6/1
  x/1 -> Product2/2

== system main_RI_LIEKF/State estimation/ER EKF/Error State Kalman Filter/Simulink Function - State Transition Jacobian ==
  DCM_b_n : Inport
  wxyz : Inport  Port=2
  fbxyz : Inport  Port=3
  stateTransitionJacobianFcn : TriggerPort  TriggerType=function-call  IsSimulinkFunction=on  FunctionName=stateTransitionJacobianFcn  VariantControl=Variant
  Cal Phi1 : Subsystem
  Constant : Constant  Value=0.01  OutDataTypeStr=single
  Data Type Conversion1 : DataTypeConversion  OutDataTypeStr=single  SaturateOnIntegerOverflow=off  RndMeth=Floor
  Data Type Conversion6 : DataTypeConversion  OutDataTypeStr=single  SaturateOnIntegerOverflow=off  RndMeth=Floor
  MATLAB Function : MATLAB Function  TreatAsAtomicUnit=on
  Terminator : Terminator
  Terminator1 : Terminator
  Transpose : Math  Operator=transpose
  x : ArgIn  DisableCoverage=on  OutDataTypeStr=single  PortDimensions=15  ArgumentName=x
  w : ArgIn  Port=2  OutDataTypeStr=single  PortDimensions=12  ArgumentName=w
  A : ArgOut  DisableCoverage=on  OutDataTypeStr=single  PortDimensions=[15 15]  ArgumentName=A
  G : ArgOut  Port=2  OutDataTypeStr=single  PortDimensions=[15 12]  ArgumentName=G
  wires:
  Data Type Conversion1/1 -> G/1
  Data Type Conversion6/1 -> A/1
  Constant/1 -> MATLAB Function/3(dt)
  Transpose/1 -> MATLAB Function/1(Cnb)
  [DCM_b_n] -> Transpose/1
  [wxyz] -> MATLAB Function/2(wxyz)
  [DCM_b_n] -> Cal Phi1/1(<DCM_b_n>)
  [fbxyz] -> Cal Phi1/3(axyz)
  [wxyz] -> Cal Phi1/2(wxyz)
  wxyz/1 -> [wxyz]
  fbxyz/1 -> [fbxyz]
  DCM_b_n/1 -> [DCM_b_n]
  Cal Phi1/1(Phi) -> Data Type Conversion6/1
  w/1 -> Terminator1/1
  x/1 -> Terminator/1
  MATLAB Function/1(G) -> Data Type Conversion1/1

== system main_RI_LIEKF/State estimation/ER EKF/Error State Kalman Filter/Subsystem ==
  data : Inport
  Detect Change : simulink/Logic and Bit Operations/Detect Change  vinit=0  InputProcessing=Columns as channels (frame based)  OutDataTypeStr=boolean
  Detect Change1 : simulink/Logic and Bit Operations/Detect Change  vinit=0  InputProcessing=Columns as channels (frame based)  OutDataTypeStr=boolean
  From Workspace1 : FromWorkspace  VariableName=[All.t',All.lat]
  From Workspace7 : FromWorkspace  Commented=on  VariableName=[All.t',All.vn]
  Selector : Selector  InputPortWidth=3  IndexOptions=Index vector (dialog)  Indices=[3]  OutputSizes=1
  Zero-Order Hold : ZeroOrderHold  SampleTime=0.2
  Zero-Order Hold1 : ZeroOrderHold  SampleTime=0.01
  flag : Outport
  wires:
  Zero-Order Hold/1 -> Selector/1
  data/1 -> Zero-Order Hold/1
  Selector/1 -> Zero-Order Hold1/1
  Detect Change1/1 -> flag/1
  Zero-Order Hold1/1 -> Detect Change/1
  From Workspace1/1 -> Detect Change1/1  "lat"

== system main_RI_LIEKF/State estimation/ER EKF/INS propogation/Init_PVQ ==
  QGC_sensor_reinit : Inport
  accl_B_m/s2_LPF : Inport  Port=2
  Magn_B_guess_LPF : Inport  Port=3
  pos_NED : Inport  Port=4
  vel_NED : Inport  Port=5
  Add : Sum
  Add1 : Sum
  Constant : Constant  Value=[0 0 0 1]  OutDataTypeStr=single
  Constant1 : Constant  OutDataTypeStr=uint8
  Constant2 : Constant  Value=[0;0;0]  OutDataTypeStr=single
  Constant3 : Constant  Value=[0;0;0]  OutDataTypeStr=single
  Constant4 : Constant  Value=[vn0;ve0;vd0]  OutDataTypeStr=single
  Constant5 : Constant  Value=[pn0;pe0;pd0]  OutDataTypeStr=single
  Detect Increase : simulink/Logic and Bit Operations/Detect Increase  vinit=0.0  OutDataTypeStr=boolean
  Horizontal_attitude : Subsystem  TreatAsAtomicUnit=on
  Horizontal_attitude2 : Subsystem  Commented=on  TreatAsAtomicUnit=on
  Memory : Memory
  Scope : Scope  NumInputPorts=2
  Scope1 : Scope
  Scope2 : Scope
  Subsystem : Subsystem
  Subsystem1 : Subsystem
  Switch{,1..3} (4 alike) : Switch  Criteria=u2 > Threshold  SaturateOnIntegerOverflow=off  InputSameDT=off
  quat_0 : Outport
  v0 : Outport  Port=2
  p0 : Outport  Port=3
  wires:
  Subsystem1/1(mean_data) -> Horizontal_attitude/2(Magn_mean_B_guess_LPF)
  Subsystem/1(mean_data) -> Horizontal_attitude/1(accl_mean_B_m/s_LPF)
  Memory/1 -> Switch1/3
  Constant/1 -> Switch/3
  Horizontal_attitude/1(quat_0) -> Switch/1
  Constant1/1 -> Switch1/1
  Switch1/1 -> Memory/1, Switch2/2, Switch3/2, Switch/2, Scope1/1
  accl_B_m/s2_LPF/1 -> Subsystem/1(data)
  QGC_sensor_reinit/1 -> Detect Increase/1, Scope/1
  Magn_B_guess_LPF/1 -> Subsystem1/1(data)
  Detect Increase/1 -> Horizontal_attitude/Enable, Switch1/2, Scope/2
  Constant2/1 -> Switch2/3
  Constant3/1 -> Switch3/3
  Switch2/1 -> v0/1
  Switch3/1 -> p0/1
  Add1/1 -> Switch3/1
  Switch/1 -> Scope2/1, quat_0/1
  Constant4/1 -> Add/2
  vel_NED/1 -> Add/1
  Add/1 -> Switch2/1
  pos_NED/1 -> Add1/1
  Constant5/1 -> Add1/2

== system main_RI_LIEKF/State estimation/ER EKF/INS propogation/accl bias compensation ==
  raw <accl_B_m/s2_LPF> : Inport
  dda : Inport  Port=2
  Add2 : Sum
  Data Type Conversion6 : DataTypeConversion  OutDataTypeStr=single  SaturateOnIntegerOverflow=off  RndMeth=Floor
  error compensation1 : Subsystem
  fb : Outport  PortDimensions=3
  da : Outport  Port=2  PortDimensions=3
  wires:
  error compensation1/1(da) -> da/1, Add2/2
  Add2/1 -> Data Type Conversion6/1
  Data Type Conversion6/1 -> fb/1
  raw <accl_B_m/s2_LPF>/1 -> Add2/1
  dda/1 -> error compensation1/1(dda)

== system main_RI_LIEKF/State estimation/ER EKF/INS propogation/att_update ==
  dtheta : Inport
  gyro : Inport  Port=2
  quat_0 : Inport  Port=3  PortDimensions=4
  init_flag : Inport  Port=4
  Bus Creator : BusCreator  Inputs=2
  Data Type Conversion1 : DataTypeConversion  OutDataTypeStr=single  SaturateOnIntegerOverflow=off  RndMeth=Floor
  Data Type Conversion2 : DataTypeConversion  OutDataTypeStr=single  SaturateOnIntegerOverflow=off  RndMeth=Floor
  Data Type Conversion3 : DataTypeConversion  OutDataTypeStr=double  SaturateOnIntegerOverflow=off  RndMeth=Floor
  Data Type Conversion4 : DataTypeConversion  OutDataTypeStr=double  SaturateOnIntegerOverflow=off  RndMeth=Floor
  Delay : Delay  DelayLength=1  InitialConditionSource=Input port  ExternalReset=Level hold
      settings: InputPortMap=u0,r5,p4
  Detect Increase : simulink/Logic and Bit Operations/Detect Increase  vinit=0.0  OutDataTypeStr=boolean
  Gain : Gain  Gain=dt  OutDataTypeStr=double
  Gain1 : Gain  Gain=-1
  JPLQuatMult : MATLAB Function  TreatAsAtomicUnit=on
  JPLQuatMult1 : MATLAB Function  TreatAsAtomicUnit=on
  JPLrv2q : MATLAB Function  TreatAsAtomicUnit=on
  JPLrv2q1 : MATLAB Function  TreatAsAtomicUnit=on
  MATLAB Function1 : MATLAB Function  TreatAsAtomicUnit=on
  Scope : Scope
  Transpose1 : Math  Operator=transpose  SignedPower=on
  att_update : Outport
  wires:
  JPLQuatMult/1(q_t) -> JPLQuatMult1/2(quatB)  "q_update"
  Detect Increase/1 -> Delay/2
  init_flag/1 -> Detect Increase/1
  Bus Creator/1 -> att_update/1
  Data Type Conversion2/1 -> Transpose1/1  "DCM_n_b"
  MATLAB Function1/1(Rot) -> Data Type Conversion2/1
  quat_0/1 -> Delay/3
  Delay/1 -> JPLQuatMult/2(quatB)
  Gain/1 -> JPLrv2q/1(rotVec)  "correctedDelAng"
  JPLrv2q/1(quaternion) -> JPLQuatMult/1(quatA)
  Data Type Conversion1/1 -> Bus Creator/1  "q_update"
  Data Type Conversion3/1 -> MATLAB Function1/1(q), Delay/1, Data Type Conversion1/1  "q_update"
  gyro/1 -> Gain/1
  Transpose1/1 -> Bus Creator/2  "DCM_b_n"
  Data Type Conversion4/1 -> JPLrv2q1/1(deltaTheta)  "q_update"
  JPLrv2q1/1(updateQuat) -> JPLQuatMult1/1(quatA)
  dtheta/1 -> Gain1/1
  Gain1/1 -> Scope/1, Data Type Conversion4/1
  JPLQuatMult1/1(q_t) -> Data Type Conversion3/1  "q_update"

== system main_RI_LIEKF/State estimation/ER EKF/INS propogation/gyro bias compensation ==
  raw <gyro_B_rad/s_LPF> : Inport
  ddg : Inport  Port=2
  Measuemrnt Enable Flag : Inport  Port=3
  Add1 : Sum
  Data Type Conversion4 : DataTypeConversion  OutDataTypeStr=single  SaturateOnIntegerOverflow=off  RndMeth=Floor
  Scope1 : Scope
  error compensation : Subsystem
  wb : Outport  PortDimensions=3
  dg : Outport  Port=2  PortDimensions=3
  wires:
  ddg/1 -> error compensation/1(ddg)
  Add1/1 -> Data Type Conversion4/1
  Measuemrnt Enable Flag/1 -> error compensation/2(Enable)
  error compensation/1(dg) -> dg/1, Scope1/1, Add1/2
  raw <gyro_B_rad/s_LPF>/1 -> Add1/1
  Data Type Conversion4/1 -> wb/1

== system main_RI_LIEKF/State estimation/ER EKF/INS propogation/vel_pos_update ==
  <DCM_b_n> : Inport
  Ab : Inport  Port=2
  v0 : Inport  Port=3
  p0 : Inport  Port=4
  QGC_init : Inport  Port=5
  dp : Inport  Port=6
  dv : Inport  Port=7
  <DCM_b_n>1 : InportShadow
  Add : Sum
  Add1 : Sum
  Add2 : Sum
  Constant : Constant  Value=[-0.45;0;0]  OutDataTypeStr=single
  Constant1 : Constant  Value=dtDelay  OutDataTypeStr=single
  Constant2 : Constant  Value=dtDelay  OutDataTypeStr=single
  Kinematic Equation : Subsystem
  Product : Product  Multiplication=Matrix(*)
  Product1 : Product
  Product2 : Product
  QGC_init1 : InportShadow  Port=5
  pos update : Subsystem
  vel update : Subsystem
  p_k : Outport  PortDimensions=3
  V : Outport  Port=2  PortDimensions=3
  pL_k : Outport  Port=3  PortDimensions=3
  VL : Outport  Port=4  PortDimensions=3
  wires:
  <DCM_b_n>/1 -> Kinematic Equation/1(Cbn)
  Ab/1 -> Kinematic Equation/2(Ab)
  QGC_init/1 -> vel update/1(QGC_init)
  dv/1 -> vel update/3(KFState_dv)
  v0/1 -> vel update/4(v0)
  dp/1 -> pos update/2(dp)
  p0/1 -> pos update/4(p0)
  pos update/1(p_k) -> Add/1, p_k/1
  QGC_init1/1 -> pos update/3(QGC_init)
  <DCM_b_n>1/1 -> Product/1
  Constant/1 -> Product/2
  Product/1 -> Add/2
  Kinematic Equation/1(An) -> Product1/2, vel update/2(An)
  vel update/1(vel_k) -> pos update/1(vel_k), Add1/2, V/1
  Product1/1 -> Add1/1
  Product2/1 -> Add2/1
  Constant1/1 -> Product1/1
  Add2/1 -> pL_k/1
  Constant2/1 -> Product2/1
  Add1/1 -> VL/1, Product2/2
  Add/1 -> Add2/2

== system main_RI_LIEKF/State estimation/LI EKF1/Error State Kalman Filter/Cal Q1 ==
  Constant : Constant  Value=dt  OutDataTypeStr=double
  MATLAB Function1 : MATLAB Function  TreatAsAtomicUnit=on
  Qd : Outport
  wires:
  MATLAB Function1/1(Q) -> Qd/1
  Constant/1 -> MATLAB Function1/1(dt)
